simulink model "example_discrete_modeling"  (R2024a)
settings: Solver=FixedStepDiscrete  StartTime=0.0  StopTime=inf  RelTol=1e-3
libraries: dspsrcs4 x1
settings Model: Creator=Admin  LastModifiedBy=Admin

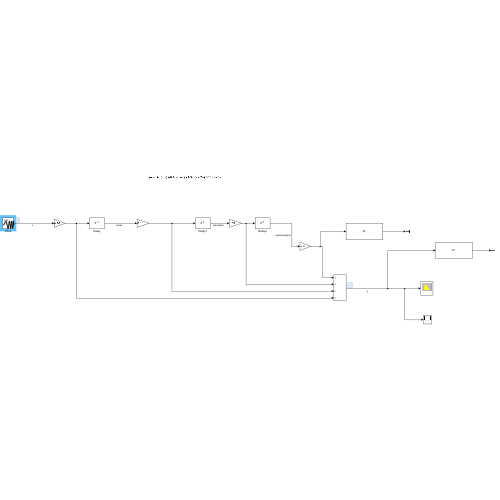
[thumbnail: Simulink's stored preview of the top-level diagram]
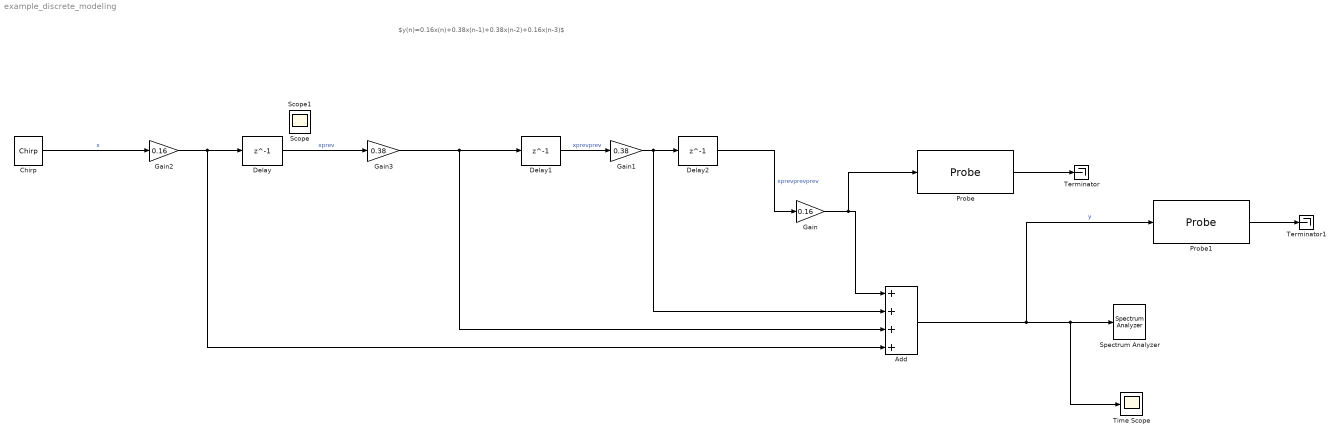
== system example_discrete_modeling ==
  note: $y(n)=0.16x(n)+0.38x(n-1)+0.38x(n-2)+0.16x(n-3)$
  Add : Sum  Inputs=++++
  Chirp : dspsrcs4/Chirp  sweep=Linear  mode=Bidirectional  f0=10  f1=4000  t1=10  Tsweep=10  phase=0  Ts=1/8000  spf=10  datatype=double  OutputFrames=off
  Delay : Delay  DelayLength=1  InitialCondition=0  UseCircularBuffer=on
  Delay1 : Delay  DelayLength=1  InitialCondition=0  UseCircularBuffer=on
  Delay2 : Delay  DelayLength=1  InitialCondition=0  UseCircularBuffer=on
  Gain : Gain  Gain=0.16
  Gain1 : Gain  Gain=0.38
  Gain2 : Gain  Gain=0.16
  Gain3 : Gain  Gain=0.38
  Probe : Probe  ProbeWidth=off  ProbeComplexSignal=off
  Probe1 : Probe  ProbeWidth=off  ProbeComplexSignal=off
  Spectrum Analyzer : SpectrumAnalyzer  WindowPosition=[263.000000,65.000000,800.000000,500.000000,]  ScopeFrameLocation=window  YLimits=[-84.51716303,1.54438815]
  Terminator : Terminator
  Terminator1 : Terminator
  Time Scope : Scope
  Scope : Scope
  Scope1 : Scope
  wires:
  Chirp/1 -> Gain2/1  "x"
  Delay/1 -> Gain3/1  "xprev"
  Delay1/1 -> Gain1/1  "xprevprev"
  Delay2/1 -> Gain/1  "xprevprevprev"
  Gain1/1 -> Add/2, Delay2/1
  Gain2/1 -> Delay/1, Add/4
  Gain3/1 -> Add/3, Delay1/1
  Gain/1 -> Probe/1, Add/1
  Add/1 -> Probe1/1, Time Scope/1, Spectrum Analyzer/1  "y"
  Probe/1 -> Terminator/1
  Probe1/1 -> Terminator1/1
